simulink model "write_control"  (R2020a)
settings: Solver=FixedStepDiscrete  StartTime=0.0  StopTime=10.0  RelTol=1e-3
settings Model: Creator=thomas  LastModifiedBy=thomas

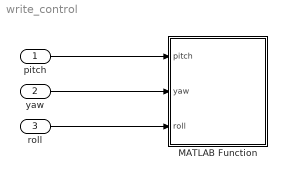
== system write_control ==
  pitch : Inport
  yaw : Inport  Port=2
  roll : Inport  Port=3
  MATLAB Function : MATLAB Function  TreatAsAtomicUnit=on
  wires:
  pitch/1 -> MATLAB Function/1(pitch)
  roll/1 -> MATLAB Function/3(roll)
  yaw/1 -> MATLAB Function/2(yaw)

== matlab function write_control/MATLAB Function ==
  data: pitch input; yaw input; roll input
function write_control(pitch, yaw, roll)
    coder.extrinsic('evalin');
    if pitch ~= 0
        evalin('base', sprintf('vessel_control.setPitch(%0.5f);', pitch));
    end
    if yaw ~= 0
        evalin('base', sprintf('vessel_control.setYaw(%0.5f);', yaw));
    end
    if roll ~= 0
        evalin('base', sprintf('vessel_control.setRoll(%0.5f);', roll));
    end
    
end
